simulink model "ATI_NetFT_nano43"  (R2016a)
settings: Solver=ode3  StartTime=0.0  StopTime=inf  FixedStep=dt  RelTol=1e-3
InitFcn:
  | PSMCMD_DEPENDENCY
  | init_NetFt
  | init_scopes
  | init_udp
  | init_resolved_rates
  | ATI_Init_nano43
  | init_LinIntPathPlan
  | init_force_control
undefined symbols (not defined in the file or in its folder): A, ATI_NetFt_reading_Gain, ATI_torque_convert_to_Nmm, dt, filter_coeffs_ATI, filter_coeffs_ATI_bias, inv_T, N_ATI, N_ATI_bias
libraries: etargetslib x9, xpcobsoletelib x3, simulink x2, dspsigops x1, xpcrtudplib x1, slrtlib x1
settings Model: Creator=Andrea  LastModifiedBy=Long
settings SolverCC: EnableConcurrentExecution=on
settings DataIOCC: LimitDataPoints=on  SaveFormat=Array  SignalLoggingSaveFormat=ModelDataLogs
settings OptimizationCC: BlockReduction=off  OptimizeBlockIOStorage=off  BufferReuse=off  GlobalBufferReuse=off  ExpressionFolding=off  ExpressionDepthLimit=2147483647  LocalBlockOutputs=off  OptimizeModelRefInitCode=on
settings DebuggingCC: UnderspecifiedInitializationDetection=Classic  MergeDetectMultiDrivingBlocksExec=none  SolverPrmCheckMsg=warning  MultiTaskCondExecSysMsg=warning  MultiTaskRateTransMsg=warning  FcnCallInpInsideContextMsg=UseLocalSettings  StateNameClashWarn=warning
settings HardwareCC: ProdBitPerPointer=32  ProdLargestAtomicFloat=None  ProdWordSize=32  ProdLongLongMode=on  ProdHWDeviceType=Generic->32-bit x86 compatible
settings ModelReferenceCC: PropagateSignalLabelsOutOfModel=off
settings SFSimCC: SimParseCustomCode=off
settings RTWCC: SystemTargetFile=slrtert.tlc  TemplateMakefile=slrtert_default_tmf  Description=Simulink Real-Time (ERT)  RTWCompilerOptimization=on
settings CodeAppCC: CustomSymbolStrType=$N$R$M  InternalIdentifier=Classic
settings SimulinkRealTimeERTCC: TargetFcnLib=ansi_tfl_table_tmw.mat  GenFloatMathFcnCalls=NOT IN USE  TargetLangStandard=C89/C90 (ANSI)  CodeReplacementLibrary=XPC_BLAS  UtilityFuncGeneration=Auto  ERTMultiwordTypeDef=System defined  ERTMultiwordLength=256  MultiwordLength=2048  GenerateFullHeader=on  InferredTypesCompatibility=off  GenerateSampleERTMain=off  GenerateTestInterfaces=off  ModelReferenceCompliant=on  ParMdlRefBuildCompliant=on  CompOptLevelCompliant=on  ConcurrentExecutionCompliant=on  IncludeMdlTerminateFcn=on  GeneratePreprocessorConditionals=Disable all  CombineOutputUpdateFcns=off  CombineSignalStateStructs=off  SuppressErrorStatus=off  ERTFirstTimeCompliant=off  IncludeFileDelimiter=Auto  ERTCustomFileBanners=off  SupportAbsoluteTime=on  LogVarNameModifier=rt_  MatFileLogging=on  MultiInstanceERTCode=off  CodeInterfacePackaging=Nonreusable function  SupportNonFinite=on  SupportComplex=on  PurelyIntegerCode=off  SupportContinuousTime=on  SupportNonInlinedSFcns=on  SupportVariableSizeSignals=off  ParenthesesLevel=Nominal  CastingMode=Nominal  MATLABClassNameForMDSCustomization=xpcAperiodicCustomization  ModelStepFunctionPrototypeControlCompliant=off  CPPClassGenCompliant=off  AutosarCompliant=off  GRTInterface=on  GenerateAllocFcn=off  UseToolchainInfoCompliant=off  GenerateSharedConstants=on  ExtModeTransport=0  ExtModeStaticAlloc=off  ExtModeStaticAllocSize=1000000  ExtModeTesting=off  InlinedParameterPlacement=Hierarchical  TargetOS=BareBoardExample  MultiInstanceErrorCode=Error  RateGroupingCode=on  RootIOFormat=Individual arguments  RTWCAPIRootIO=off  EnableDataOwnership=off  ERTFilePackagingFormat=Modular  PreserveExpressionOrder=off  PreserveIfCondition=off  ConvertIfToSwitch=off  PreserveExternInFcnDecls=on  SuppressUnreachableDefaultCases=off  EnableSignedLeftShifts=on  EnableSignedRightShifts=on  IndentStyle=K&R  IndentSize=2  EnableUserReplacementTypes=off  MaxIdInt32=MAX_int32_T  MinIdInt32=MIN_int32_T  MaxIdUint32=MAX_uint32_T  MaxIdInt16=MAX_int16_T  MinIdInt16=MIN_int16_T  MaxIdUint16=MAX_uint16_T  MaxIdInt8=MAX_int8_T  MinIdInt8=MIN_int8_T  MaxIdUint8=MAX_uint8_T  BooleanTrueId=true  BooleanFalseId=false  MemSecPackage=--- None ---  MemSecDataConstants=Default  MemSecDataIO=Default  MemSecDataInternal=Default  MemSecDataParameters=Default  MemSecFuncInitTerm=Default  MemSecFuncExecute=Default  MemSecFuncSharedUtil=Default  GlobalDataDefinition=Auto  GlobalDataReference=Auto  GenerateASAP2=off  ERTSrcFileBannerTemplate=ert_code_template.cgt  ERTHdrFileBannerTemplate=ert_code_template.cgt  ERTDataSrcFileTemplate=ert_code_template.cgt  ERTDataHdrFileTemplate=ert_code_template.cgt  ERTCustomFileTemplate=example_file_process.tlc  SignalDisplayLevel=10  ParamTuneLevel=10  InitialValueSource=Model  RTWCAPISignals=off  RTWCAPIParams=on  RTWCAPIStates=off  RL32ModeModifier=Real-Time  ExtMode=on  ExtModeMexFile=ext_xpc  ExtModeIntrfLevel=Level2 - Open  ExtModeArmWhenConnect=off  RL32LogTETModifier=on  RL32LogBufSizeModifier=100000  xPCTaskExecutionProfile=off  xPCRL32EventNumber=5000  RL32IRQSourceModifier=Timer  xPCIRQSourceBoard=None/Other  xPCIOIRQSlot=-1  xpcObjCom=off  xPCGenerateASAP2=off  xPCGenerateXML=off  RL32ObjectName=tg  xPCisDownloadable=off  xPCisDefaultEnv=on  xPCisModelTimeout=on  xPCModelTimeoutSecs=5  xpcDblBuff=off  xPCLoadParamSetFile=off  xPCConcurrentTasks=off  xPCEnableSFAnimation=off
settings ConfigComp: CovModelRefEnable=Off

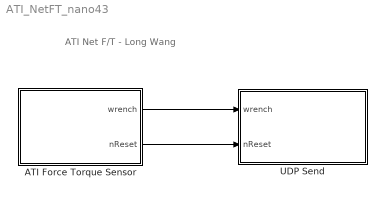
== system ATI_NetFT_nano43 ==
  note: ATI Net F/T - Long Wang
  ATI Force Torque Sensor : Subsystem
  UDP Send : Subsystem
  wires:
  ATI Force Torque Sensor/1(wrench) -> UDP Send/1(wrench)
  ATI Force Torque Sensor/2(nReset) -> UDP Send/2(nReset)

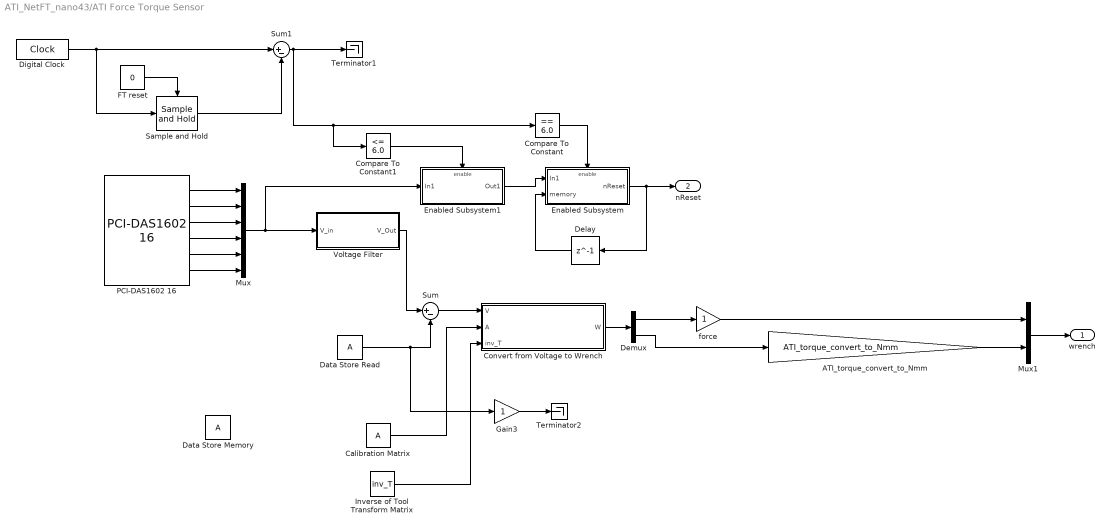
== system ATI_NetFT_nano43/ATI Force Torque Sensor ==
  ATI_torque_convert_to_Nmm : Gain  Gain=ATI_torque_convert_to_Nmm
  Calibration Matrix : Constant  Value=A
  Compare To Constant : simulink/Logic and Bit Operations/Compare To Constant  relop===  const=6.0  OutDataTypeStr=uint8  ZeroCross=off
  Compare To Constant1 : simulink/Logic and Bit Operations/Compare To Constant  relop=<=  const=6.0  OutDataTypeStr=uint8  ZeroCross=off
  "Convert from Voltage to Wrench " : MATLAB Function  TreatAsAtomicUnit=on
  Data Store Memory : DataStoreMemory  ReadBeforeWriteMsg=warning  WriteAfterWriteMsg=warning  WriteAfterReadMsg=warning  InitialValue=[0;0;0;0;0;0]  ShowAdditionalParam=off
  Data Store Read : DataStoreRead  SampleTime=0
  Delay : Delay  DelayLength=1  InitialCondition=0
  Demux : Demux  Outputs=2
  Digital Clock : DigitalClock  SampleTime=dt
  Enabled Subsystem : Subsystem  TreatAsAtomicUnit=on
  Enabled Subsystem1 : Subsystem  TreatAsAtomicUnit=on
  FT reset : Constant  Value=0
  Gain3 : Gain
  Inverse of Tool Transform Matrix : Constant  Value=inv_T  VectorParams1D=off
  Mux : Mux  Inputs=6
  Mux1 : Mux  Inputs=2
  "PCI-DAS1602 16 " : xpcobsoletelib/Measurement Computing obs/A//D/PCI-DAS1602 16   channel=6  range=+-10V  mux=Differential (8 channels)  sampletime=dt  slot=[4 1]
  Sample and Hold : dspsigops/Sample and Hold  trig=Rising edge  initCond=0  latchinput=off
  Sum : Sum  Inputs=|+-
  Sum1 : Sum  Inputs=|+-
  Terminator1 : Terminator
  Terminator2 : Terminator
  Voltage Filter : Subsystem
  force : Gain
  wrench : Outport
  nReset : Outport  Port=2
  wires:
  Mux/1 -> Voltage Filter/1(V_in), Enabled Subsystem1/1(In1)
  Calibration Matrix/1 -> "Convert from Voltage to Wrench "/2(A)
  Inverse of Tool Transform Matrix/1 -> "Convert from Voltage to Wrench "/3(inv_T)
  Sum/1 -> "Convert from Voltage to Wrench "/1(V)
  Voltage Filter/1(V_Out) -> Sum/1
  Data Store Read/1 -> Sum/2, Gain3/1
  Enabled Subsystem1/1(Out1) -> Enabled Subsystem/1(In1)
  Compare To Constant/1 -> Enabled Subsystem/Enable
  Gain3/1 -> Terminator2/1
  Compare To Constant1/1 -> Enabled Subsystem1/Enable
  "PCI-DAS1602 16 "/1 -> Mux/1
  "PCI-DAS1602 16 "/2 -> Mux/2
  "PCI-DAS1602 16 "/3 -> Mux/3
  "PCI-DAS1602 16 "/4 -> Mux/4
  "PCI-DAS1602 16 "/5 -> Mux/5
  "PCI-DAS1602 16 "/6 -> Mux/6
  Digital Clock/1 -> Sum1/1, Sample and Hold/1
  Sum1/1 -> Terminator1/1, Compare To Constant/1, Compare To Constant1/1
  Sample and Hold/1 -> Sum1/2
  FT reset/1 -> Sample and Hold/Trigger
  Demux/1 -> force/1
  Demux/2 -> ATI_torque_convert_to_Nmm/1
  ATI_torque_convert_to_Nmm/1 -> Mux1/2
  "Convert from Voltage to Wrench "/1(W) -> Demux/1
  force/1 -> Mux1/1
  Mux1/1 -> wrench/1
  Enabled Subsystem/1(nReset) -> Delay/1, nReset/1
  Delay/1 -> Enabled Subsystem/2(memory)

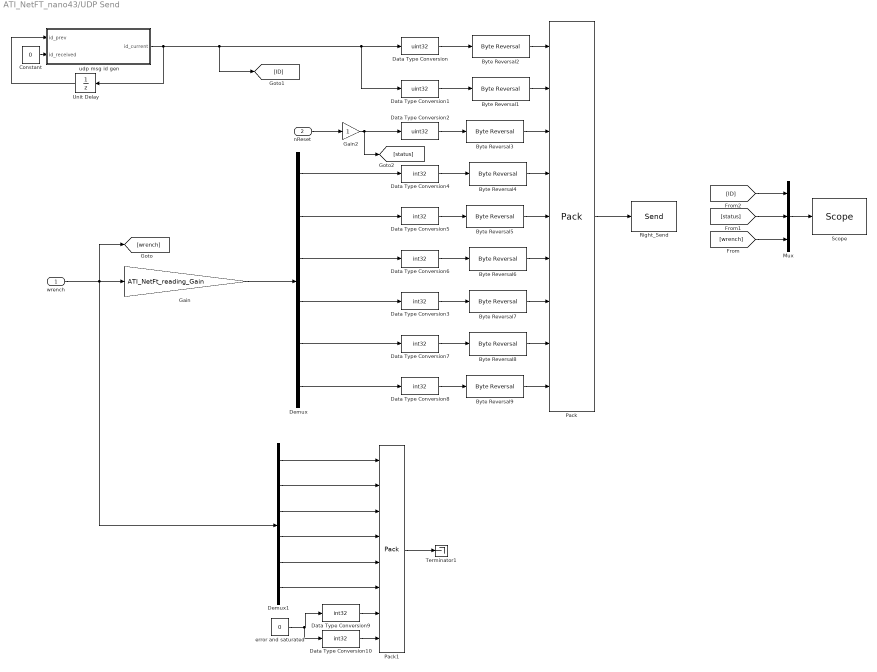
== system ATI_NetFT_nano43/UDP Send ==
  wrench : Inport
  nReset : Inport  Port=2
  Byte Reversal{1..9} (9 alike) : etargetslib/Byte Reversal  numInp=1
  Constant : Constant  Value=0
  Data Type Conversion : DataTypeConversion  OutDataTypeStr=uint32
  Data Type Conversion1 : DataTypeConversion  OutDataTypeStr=uint32
  Data Type Conversion{3..10} (8 alike) : DataTypeConversion  OutDataTypeStr=int32
  Data Type Conversion2 : DataTypeConversion  OutDataTypeStr=uint32  RndMeth=Nearest
  Demux : Demux  Outputs=6
  Demux1 : Demux  Outputs=6
  Gain : Gain  Gain=ATI_NetFt_reading_Gain
  Gain2 : Gain
  Mux : Mux  Inputs=[1,1,6]
  Pack : xpcobsoletelib/Utilities/Pack   datatypes=socketSentFtMsgTypes  byteAlign=1
  Pack1 : xpcobsoletelib/Utilities/Pack   datatypes={'double' 'double' 'double' 'double' 'double' 'double' 'int32' 'int32'}  byteAlign=1
  Right_Send : xpcrtudplib/Legacy UDP/Send   ipAddress=192.168.1.201  ipPort=ATI_NetFt_port  localPort=-1  vblLen=off  sampletime=dt_udp
  "Scope " : slrtlib/Displays and Logging/Scope   scopeno=9  scopetype=Target  autostart=on  viewmode=Numerical  formatstr=Scope_format_socketSentFtMsg  grid=on  ylimits=[0,0]  nosamples=10  noprepostsamples=0  interleave=1  triggermode=FreeRun  triggersignal=1  trigsignalfromport=off  triggerlevel=0.0  triggerslope=Either  triggerscope=1  triggersample=0  filename=data.dat  mode=Lazy  writesize=512  autorestart=off  dynamicfilemode=off  maxwritefilesize=512*1024^2
  Terminator1 : Terminator
  Unit Delay : UnitDelay  SampleTime=-1
  error and saturated : Constant  Value=0  VectorParams1D=off
  udp msg id gen : MATLAB Function  TreatAsAtomicUnit=on
  wires:
  Demux/1 -> Data Type Conversion4/1
  Demux/4 -> Data Type Conversion3/1
  Demux/5 -> Data Type Conversion7/1
  Demux/3 -> Data Type Conversion6/1
  Demux/2 -> Data Type Conversion5/1
  Demux/6 -> Data Type Conversion8/1
  nReset/1 -> Gain2/1
  Data Type Conversion8/1 -> Byte Reversal9/1
  Data Type Conversion5/1 -> Byte Reversal5/1
  Data Type Conversion/1 -> Byte Reversal2/1
  Data Type Conversion2/1 -> Byte Reversal3/1
  Data Type Conversion6/1 -> Byte Reversal6/1
  Data Type Conversion7/1 -> Byte Reversal8/1
  Data Type Conversion4/1 -> Byte Reversal4/1
  Data Type Conversion1/1 -> Byte Reversal1/1
  Data Type Conversion3/1 -> Byte Reversal7/1
  Unit Delay/1 -> udp msg id gen/1(id_prev)
  Constant/1 -> udp msg id gen/2(id_received)
  wrench/1 -> Demux1/1, [wrench], Gain/1
  Gain/1 -> Demux/1
  udp msg id gen/1(id_current) -> [ID], Data Type Conversion1/1, Data Type Conversion/1, Unit Delay/1
  Mux/1 -> "Scope "/1
  [wrench] -> Mux/3
  [ID] -> Mux/1
  Gain2/1 -> [status], Data Type Conversion2/1
  [status] -> Mux/2
  Pack/1 -> Right_Send/1
  Demux1/2 -> Pack1/2
  Demux1/4 -> Pack1/4
  Demux1/3 -> Pack1/3
  Demux1/5 -> Pack1/5
  Demux1/6 -> Pack1/6
  Demux1/1 -> Pack1/1
  Data Type Conversion9/1 -> Pack1/7
  Data Type Conversion10/1 -> Pack1/8
  error and saturated/1 -> Data Type Conversion10/1, Data Type Conversion9/1
  Pack1/1 -> Terminator1/1
  Byte Reversal2/1 -> Pack/1
  Byte Reversal1/1 -> Pack/2
  Byte Reversal3/1 -> Pack/3
  Byte Reversal4/1 -> Pack/4
  Byte Reversal5/1 -> Pack/5
  Byte Reversal6/1 -> Pack/6
  Byte Reversal7/1 -> Pack/7
  Byte Reversal8/1 -> Pack/8
  Byte Reversal9/1 -> Pack/9

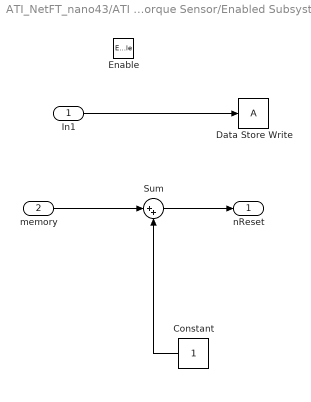
== system ATI_NetFT_nano43/ATI Force Torque Sensor/Enabled Subsystem ==
  In1 : Inport
  memory : Inport  Port=2
  Enable : EnablePort
  Constant : Constant
  Data Store Write : DataStoreWrite
  Sum : Sum  Inputs=|++
  nReset : Outport  InitialOutput=0
  wires:
  In1/1 -> Data Store Write/1
  Constant/1 -> Sum/2
  memory/1 -> Sum/1
  Sum/1 -> nReset/1

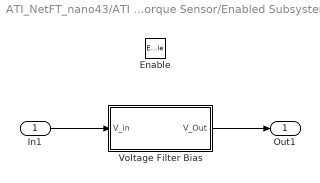
== system ATI_NetFT_nano43/ATI Force Torque Sensor/Enabled Subsystem1 ==
  In1 : Inport
  Enable : EnablePort
  Voltage Filter Bias : Subsystem
  Out1 : Outport
  wires:
  In1/1 -> Voltage Filter Bias/1(V_in)
  Voltage Filter Bias/1(V_Out) -> Out1/1

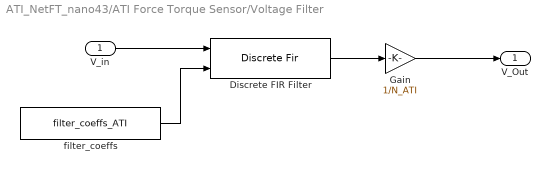
== system ATI_NetFT_nano43/ATI Force Torque Sensor/Voltage Filter ==
  V_in : Inport
  Discrete FIR Filter : DiscreteFir  CoefSource=Input port  AccumDataTypeStr=Inherit: Same as product output
      settings: InputPortMap=u0,u1
  Gain : Gain  Gain=1/N_ATI
  filter_coeffs : Constant  Value=filter_coeffs_ATI
  V_Out : Outport
  wires:
  V_in/1 -> Discrete FIR Filter/1
  Discrete FIR Filter/1 -> Gain/1
  filter_coeffs/1 -> Discrete FIR Filter/2
  Gain/1 -> V_Out/1

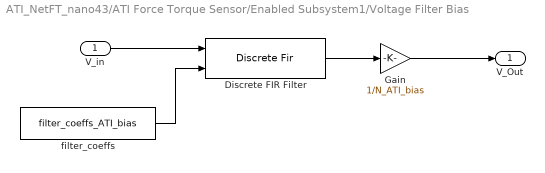
== system ATI_NetFT_nano43/ATI Force Torque Sensor/Enabled Subsystem1/Voltage Filter Bias ==
  V_in : Inport
  Discrete FIR Filter : DiscreteFir  CoefSource=Input port  AccumDataTypeStr=Inherit: Same as product output
      settings: InputPortMap=u0,u1
  Gain : Gain  Gain=1/N_ATI_bias
  filter_coeffs : Constant  Value=filter_coeffs_ATI_bias
  V_Out : Outport
  wires:
  Gain/1 -> V_Out/1
  filter_coeffs/1 -> Discrete FIR Filter/2
  Discrete FIR Filter/1 -> Gain/1
  V_in/1 -> Discrete FIR Filter/1

== matlab function ATI_NetFT_nano43/ATI Force Torque Sensor/Convert from Voltage to Wrench  ==
  data: V input; W output; A input; inv_T input
function W = Convert_Function(V,A,inv_T)%A_vec,p)

W = inv_T*A*V;

== matlab function ATI_NetFT_nano43/UDP Send/udp msg id gen ==
  data: id_prev input; id_current output; id_received input
function id_current = MsgIDGen(id_prev,id_received)
%#codegen
%%  Generate message ID
if id_received==1
    id_current = 2;
else
    id_current = id_prev + 1;
end
